simulink model "four_levels"  (R2017b)
settings: Solver=ode45  StartTime=0.0  StopTime=4  RelTol=1e-3  AbsTol=1e-6
libraries: simulink_extras x3, commsequence2 x1
settings Model: ExtModeTrigMode=oneshot  ExtModeArmWhenConnect=off  Creator=cv  LastModifiedBy=cv
settings DataIOCC: SaveFormat=Array  SignalLoggingSaveFormat=ModelDataLogs  SignalLoggingName=sigsOut
settings OptimizationCC: BooleanDataType=off  InitFltsAndDblsToZero=on  LifeSpan=inf
settings DebuggingCC: SaveWithParameterizedLinksMsg=none  UnderspecifiedInitializationDetection=Classic  MergeDetectMultiDrivingBlocksExec=none  SignalResolutionControl=TryResolveAllWithWarning  MultiTaskDSMMsg=warning  MultiTaskCondExecSysMsg=none  FcnCallInpInsideContextMsg=warning  StrictBusMsg=None  SFUnexpectedBacktrackingDiag=warning  SFNoUnconditionalDefaultTransitionDiag=warning  SFExecutionAtInitializationDiag=none
settings HardwareCC: ProdBitPerPointer=32  ProdBitPerSizeT=32  ProdBitPerPtrDiffT=32  ProdLargestAtomicFloat=None  ProdIntDivRoundTo=Undefined  ProdEndianess=Unspecified  ProdWordSize=32  ProdHWDeviceType=32-bit Generic  TargetUnknown=on
settings ModelReferenceCC: PropagateSignalLabelsOutOfModel=off
settings RTWCC: Description=Generic Real-Time Target
settings CodeAppCC: StateflowObjectComments=on
settings GRTTargetCC: TargetFcnLib=ansi_tfl_tmw.mat  TargetLangStandard=C89/C90 (ANSI)  CombineOutputUpdateFcns=off  GRTInterface=on
settings ConfigComp: CovMetricSettings=dw  CovHtmlReporting=on  CovSaveCumulativeToWorkspaceVar=on  CovSaveSingleToWorkspaceVar=on  CovExternalEMLEnable=off

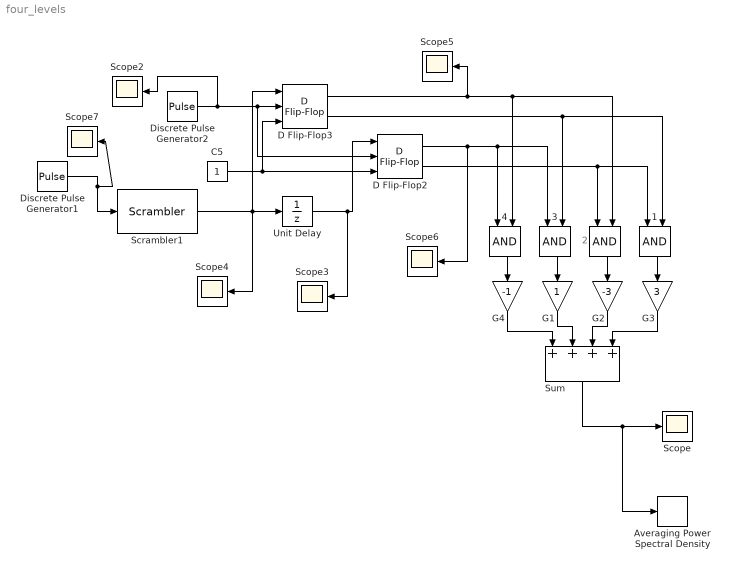
== system four_levels ==
  note: 2
  " " : Logic
  " 1" : Logic
  3 : Logic
  4 : Logic
  Averaging Power Spectral Density : simulink_extras/Additional Sinks/Averaging Power Spectral Density  npts=512  fftpts=4096  HowOften=256  sampleT=2*pi/30000
      link override sfunpsd: FunctionName=sfunpsd_mod  Parameters=fftpts,npts,HowOften,offset,ts,1,type_disp
      settings: SourceProductName=Simulink  SourceProductBaseCode=SL
  C5 : Constant
  D Flip-Flop2 : simulink_extras/Flip Flops/D Flip-Flop
      settings: SourceProductName=Simulink
  D Flip-Flop3 : simulink_extras/Flip Flops/D Flip-Flop
      settings: SourceProductName=Simulink
  Discrete Pulse Generator1 : DiscretePulseGenerator  Period=8  SampleTime=2*pi/10000
      settings: AttributesFormatString=1:7
  Discrete Pulse Generator2 : DiscretePulseGenerator  Period=4  PhaseDelay=2  SampleTime=2*pi/20000
      settings: AttributesFormatString=1:5
  G1 : Gain  SaturateOnIntegerOverflow=on  OutDataTypeStr=Inherit: Same as input  ParamDataTypeStr=Inherit: Same as input
  G2 : Gain  Gain=-3  SaturateOnIntegerOverflow=on  OutDataTypeStr=Inherit: Same as input  ParamDataTypeStr=Inherit: Same as input
  G3 : Gain  Gain=3  SaturateOnIntegerOverflow=on  OutDataTypeStr=Inherit: Same as input  ParamDataTypeStr=Inherit: Same as input
  G4 : Gain  Gain=-1  SaturateOnIntegerOverflow=on  OutDataTypeStr=Inherit: Same as input  ParamDataTypeStr=Inherit: Same as input
  Scope{,2..7} (7 alike) : Scope
  Scrambler1 : commsequence2/Scrambler  M=2  poly=[0 -1 -7]  iniStaSource=Dialog Parameter  ini_sta=[1 1 1 1 1 1 1]  resetViaPort=off
      settings: SourceProductName=Communications System Toolbox  SourceProductBaseCode=CM
  Sum : Sum  Inputs=++++  SaturateOnIntegerOverflow=on  InputSameDT=on  OutDataTypeStr=Inherit: Same as first input
  Unit Delay : UnitDelay  InitialCondition=1  SampleTime=-1
  wires:
  C5/1 -> D Flip-Flop3/3, D Flip-Flop2/3
  Scrambler1/1 -> D Flip-Flop3/1, Unit Delay/1, Scope4/1
  D Flip-Flop2/2 -> " 1"/1, " "/1
  D Flip-Flop3/2 -> " 1"/2, 3/2
  " 1"/1 -> G3/1
  3/1 -> G1/1
  " "/1 -> G2/1
  G1/1 -> Sum/2
  G2/1 -> Sum/3
  G3/1 -> Sum/4
  Discrete Pulse Generator2/1 -> D Flip-Flop3/2, D Flip-Flop2/2, Scope2/1
  Unit Delay/1 -> D Flip-Flop2/1, Scope3/1
  D Flip-Flop3/1 -> " "/2, 4/2, Scope5/1
  D Flip-Flop2/1 -> 3/1, 4/1, Scope6/1
  Discrete Pulse Generator1/1 -> Scope7/1, Scrambler1/1
  4/1 -> G4/1
  G4/1 -> Sum/1
  Sum/1 -> Scope/1, Averaging Power Spectral Density/1
